simulink model "htx_intent_estimator_base"  (R2024b)
settings: Solver=VariableStepAuto  StartTime=0.0  StopTime=1  FixedStep=0.001  RelTol=1e-3
libraries: simulink_extras x1
settings Model: Creator=lukec  LastModifiedBy=lukec
settings SolverCC: ZeroCrossControl=DisableAll

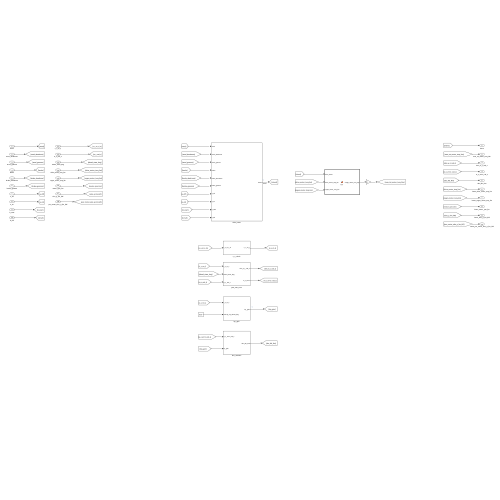
[thumbnail: Simulink's stored preview of the top-level diagram]
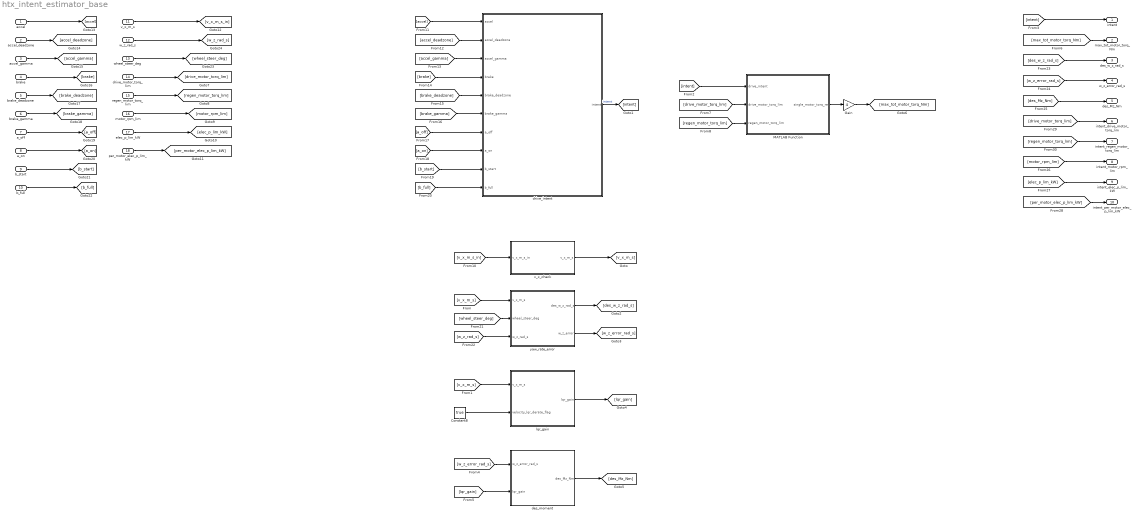
== system htx_intent_estimator_base ==
  accel : Inport
  accel_deadzone : Inport  Port=2
  accel_gamma : Inport  Port=3
  brake : Inport  Port=4
  brake_deadzone : Inport  Port=5
  brake_gamma : Inport  Port=6
  a_off : Inport  Port=7
  a_on : Inport  Port=8
  b_start : Inport  Port=9
  b_full : Inport  Port=10
  v_x_m_s : Inport  Port=11
  w_z_rad_s : Inport  Port=12
  wheel_steer_deg : Inport  Port=13
  drive_motor_torq_lim : Inport  Port=14
  regen_motor_torq_lim : Inport  Port=15
  motor_rpm_lim : Inport  Port=16
  elec_p_lim_kW : Inport  Port=17
  per_motor_elec_p_lim_kW : Inport  Port=18
  Constant8 : Constant  Value=true
  Gain : Gain  Gain=4
  MATLAB Function : MATLAB Function  TreatAsAtomicUnit=on
  des_moment : Subsystem
  drive_intent : Subsystem
  lqr_gain : Subsystem
  v_x_check : Subsystem
  yaw_rate_error : Subsystem
  intent : Outport
  max_tot_motor_torq_Nm : Outport  Port=2
  des_w_z_rad_s : Outport  Port=3
  w_z_error_rad_s : Outport  Port=4
  des_Mz_Nm : Outport  Port=5
  intent_drive_motor_torq_lim : Outport  Port=6
  intent_regen_motor_torq_lim : Outport  Port=7
  intent_motor_rpm_lim : Outport  Port=8
  intent_elec_p_lim_kW : Outport  Port=9
  intent_per_motor_elec_p_lim_kW : Outport  Port=10
  wires:
  Constant8/1 -> lqr_gain/2(velocity_lqr_derate_flag)
  lqr_gain/1(lqr_gain) -> [lqr_gain]
  [v_x_m_s] -> yaw_rate_error/1(v_x_m_s)
  [v_x_m_s] -> lqr_gain/1(v_x_m_s)
  MATLAB Function/1(single_motor_torq_req) -> Gain/1
  drive_intent/1(intent) -> [intent]  "intent"
  [intent] -> MATLAB Function/1(drive_intent)
  [intent] -> intent/1
  yaw_rate_error/1(des_w_z_rad_s) -> [des_w_z_rad_s]
  yaw_rate_error/2(w_z_error) -> [w_z_error_rad_s]
  [w_z_error_rad_s] -> des_moment/1(w_z_error_rad_s)
  [lqr_gain] -> des_moment/2(lqr_gain)
  des_moment/1(des_Mz_Nm) -> [des_Mz_Nm]
  Gain/1 -> [max_tot_motor_torq_Nm]
  [max_tot_motor_torq_Nm] -> max_tot_motor_torq_Nm/1
  regen_motor_torq_lim/1 -> [regen_motor_torq_lim]
  drive_motor_torq_lim/1 -> [drive_motor_torq_lim]
  [drive_motor_torq_lim] -> MATLAB Function/2(drive_motor_torq_lim)
  [regen_motor_torq_lim] -> MATLAB Function/3(regen_motor_torq_lim)
  motor_rpm_lim/1 -> [motor_rpm_lim]
  elec_p_lim_kW/1 -> [elec_p_lim_kW]
  per_motor_elec_p_lim_kW/1 -> [per_motor_elec_p_lim_kW]
  v_x_m_s/1 -> [v_x_m_s_in]
  accel/1 -> [accel]
  accel_deadzone/1 -> [accel_deadzone]
  accel_gamma/1 -> [accel_gamma]
  brake/1 -> [brake]
  brake_deadzone/1 -> [brake_deadzone]
  brake_gamma/1 -> [brake_gamma]
  a_off/1 -> [a_off]
  a_on/1 -> [a_on]
  b_start/1 -> [b_start]
  b_full/1 -> [b_full]
  [accel] -> drive_intent/1(accel)
  [accel_deadzone] -> drive_intent/2(accel_deadzone)
  [accel_gamma] -> drive_intent/3(accel_gamma)
  [b_full] -> drive_intent/10(b_full)
  [b_start] -> drive_intent/9(b_start)
  [a_on] -> drive_intent/8(a_on)
  [a_off] -> drive_intent/7(a_off)
  [brake_gamma] -> drive_intent/6(brake_gamma)
  [brake_deadzone] -> drive_intent/5(brake_deadzone)
  [brake] -> drive_intent/4(brake)
  wheel_steer_deg/1 -> [wheel_steer_deg]
  w_z_rad_s/1 -> [w_z_rad_s]
  [wheel_steer_deg] -> yaw_rate_error/2(wheel_steer_deg)
  [w_z_rad_s] -> yaw_rate_error/3(w_z_rad_s)
  [des_w_z_rad_s] -> des_w_z_rad_s/1
  [w_z_error_rad_s] -> w_z_error_rad_s/1
  [des_Mz_Nm] -> des_Mz_Nm/1
  [motor_rpm_lim] -> intent_motor_rpm_lim/1
  [elec_p_lim_kW] -> intent_elec_p_lim_kW/1
  [per_motor_elec_p_lim_kW] -> intent_per_motor_elec_p_lim_kW/1
  [drive_motor_torq_lim] -> intent_drive_motor_torq_lim/1
  [regen_motor_torq_lim] -> intent_regen_motor_torq_lim/1
  [v_x_m_s_in] -> v_x_check/1(v_x_m_s_in)
  v_x_check/1(v_x_m_s) -> [v_x_m_s]

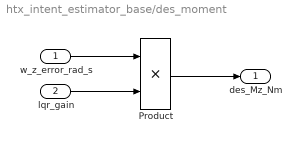
== system htx_intent_estimator_base/des_moment ==
  w_z_error_rad_s : Inport
  lqr_gain : Inport  Port=2
  Product : Product
  des_Mz_Nm : Outport
  wires:
  w_z_error_rad_s/1 -> Product/1
  lqr_gain/1 -> Product/2
  Product/1 -> des_Mz_Nm/1

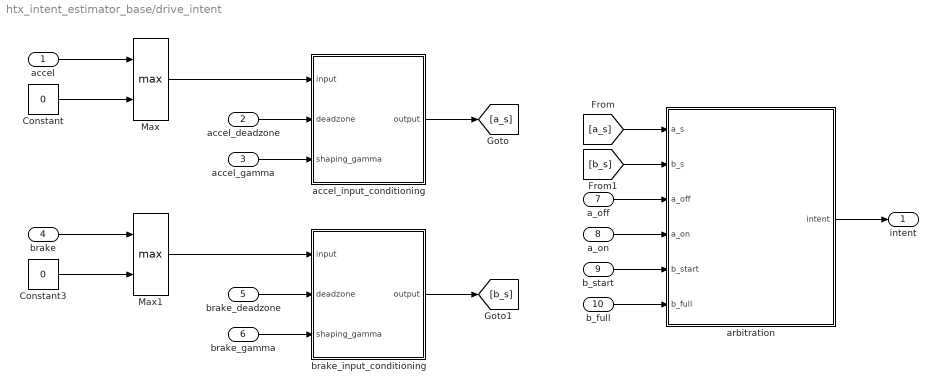
== system htx_intent_estimator_base/drive_intent ==
  accel : Inport
  accel_deadzone : Inport  Port=2
  accel_gamma : Inport  Port=3
  brake : Inport  Port=4
  brake_deadzone : Inport  Port=5
  brake_gamma : Inport  Port=6
  a_off : Inport  Port=7
  a_on : Inport  Port=8
  b_start : Inport  Port=9
  b_full : Inport  Port=10
  Constant : Constant  Value=0
  Constant3 : Constant  Value=0
  Max : MinMax  Function=max  Inputs=2
  Max1 : MinMax  Function=max  Inputs=2
  accel_input_conditioning : Subsystem
  arbitration : Subsystem
  brake_input_conditioning : Subsystem
  intent : Outport
  wires:
  accel/1 -> Max/1
  Constant/1 -> Max/2
  Max/1 -> accel_input_conditioning/1(input)
  accel_gamma/1 -> accel_input_conditioning/3(shaping_gamma)
  accel_input_conditioning/1(output) -> [a_s]
  accel_deadzone/1 -> accel_input_conditioning/2(deadzone)
  brake/1 -> Max1/1
  Constant3/1 -> Max1/2
  Max1/1 -> brake_input_conditioning/1(input)
  brake_deadzone/1 -> brake_input_conditioning/2(deadzone)
  brake_gamma/1 -> brake_input_conditioning/3(shaping_gamma)
  brake_input_conditioning/1(output) -> [b_s]
  [a_s] -> arbitration/1(a_s)
  [b_s] -> arbitration/2(b_s)
  arbitration/1(intent) -> intent/1
  a_off/1 -> arbitration/3(a_off)
  a_on/1 -> arbitration/4(a_on)
  b_start/1 -> arbitration/5(b_start)
  b_full/1 -> arbitration/6(b_full)

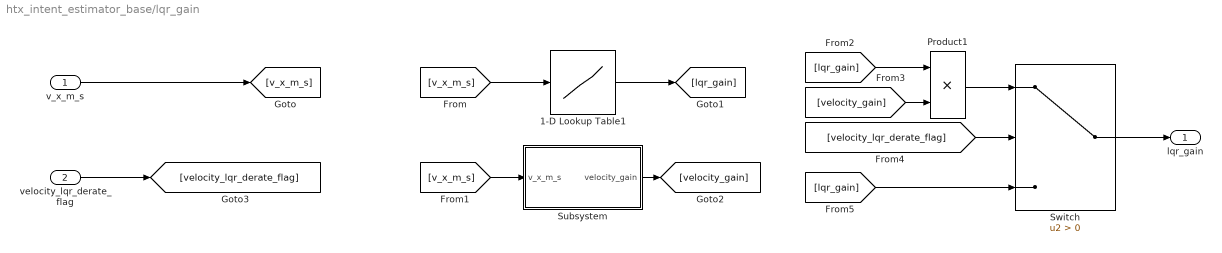
== system htx_intent_estimator_base/lqr_gain ==
  v_x_m_s : Inport
  velocity_lqr_derate_flag : Inport  Port=2
  1-D Lookup Table1 : Lookup_n-D  NumberOfTableDimensions=1  BreakpointsForDimension1="[1\t2\t3\t4\t5\t6\t7\t8\t9\t10\t11\t12\t13\t14\t15\t16\t17\t18\t19\t20\t21\t22\t23\t24\t25\t26\t27\t28\t29\t30\t31\t32\t33\t34\t35]"  Table=|  ExtrapMethod=Clip  UseLastTableValue=on  InternalRulePriority=Speed  RndMeth=Simplest
      | [175.998769578400
      | 348.795608426570
      | 515.559078921668
      | 674.093445795412
      | 822.946224394498
      | 961.371891615202
      | 1089.20563526030
      | 1206.70525770109
      | 1314.40207126520
      | 1412.98049731322
      | 1503.19064596410
      | 1585.79003907249
      | 1661.50785065425
      | 1731.02511425824
      | 1794.96555127361
      | 1853.89307906945
      | 1908.31327556636
      | 1958.67700477001
      | 2005.38506538649
      | 2048.79316923418
      | 2089.21684666341
      | 2126.93606072781
      | 2162.19942593451
      | 2195.22799578584
      | 2226.21862266091
      | 2255.34691480485
      | 2282.76982535041
      | 2308.62791187574
      | 2333.04730481808
      | 2356.14142085417
      | 2378.01245418101
      | 2398.75267510957
      | 2418.44556187634
      | 2437.16678827469
      | 2454.98508670055]
  Product1 : Product
  Subsystem : Subsystem
  Switch : Switch  Criteria=u2 > Threshold  SaturateOnIntegerOverflow=off  InputSameDT=off
  lqr_gain : Outport
  wires:
  Product1/1 -> Switch/1
  v_x_m_s/1 -> [v_x_m_s]
  [v_x_m_s] -> 1-D Lookup Table1/1
  1-D Lookup Table1/1 -> [lqr_gain]
  [v_x_m_s] -> Subsystem/1(v_x_m_s)
  Subsystem/1(velocity_gain) -> [velocity_gain]
  [lqr_gain] -> Product1/1
  [velocity_gain] -> Product1/2
  velocity_lqr_derate_flag/1 -> [velocity_lqr_derate_flag]
  [velocity_lqr_derate_flag] -> Switch/2
  [lqr_gain] -> Switch/3
  Switch/1 -> lqr_gain/1

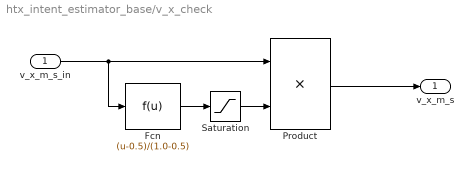
== system htx_intent_estimator_base/v_x_check ==
  v_x_m_s_in : Inport
  Fcn : Fcn  Expr=(u-0.5)/(1.0-0.5)
  Product : Product
  Saturation : Saturate  UpperLimit=1  LowerLimit=0
  v_x_m_s : Outport
  wires:
  v_x_m_s_in/1 -> Fcn/1, Product/1
  Product/1 -> v_x_m_s/1
  Fcn/1 -> Saturation/1
  Saturation/1 -> Product/2

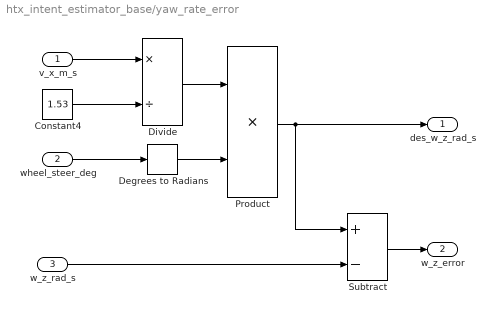
== system htx_intent_estimator_base/yaw_rate_error ==
  v_x_m_s : Inport
  wheel_steer_deg : Inport  Port=2
  w_z_rad_s : Inport  Port=3
  Constant4 : Constant  Value=1.53
  Degrees to Radians : simulink_extras/Transformations/Degrees to Radians
  Divide : Product  Inputs=*/
  Product : Product
  Subtract : Sum  Inputs=+-
  des_w_z_rad_s : Outport
  w_z_error : Outport  Port=2
  wires:
  wheel_steer_deg/1 -> Degrees to Radians/1
  Divide/1 -> Product/1
  Degrees to Radians/1 -> Product/2
  Constant4/1 -> Divide/2
  v_x_m_s/1 -> Divide/1
  Product/1 -> des_w_z_rad_s/1, Subtract/1
  w_z_rad_s/1 -> Subtract/2
  Subtract/1 -> w_z_error/1

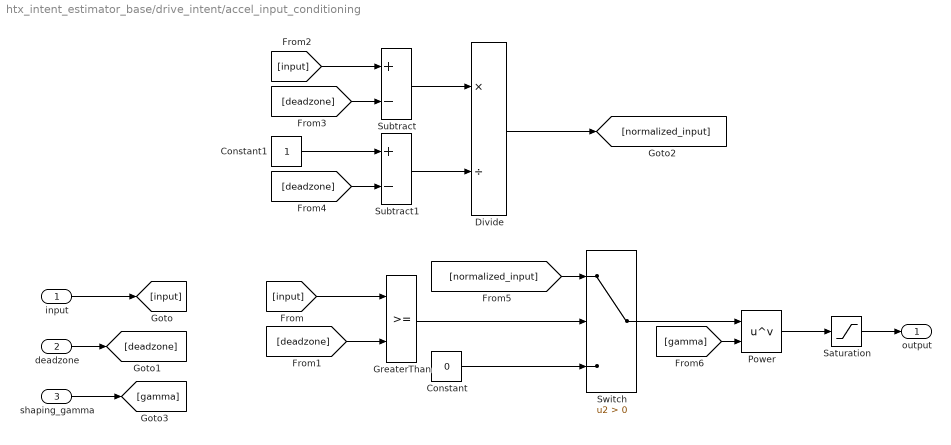
== system htx_intent_estimator_base/drive_intent/accel_input_conditioning ==
  input : Inport
  deadzone : Inport  Port=2
  shaping_gamma : Inport  Port=3
  Constant : Constant  Value=0
  Constant1 : Constant
  Divide : Product  Inputs=*/
  GreaterThan : RelationalOperator  OutDataTypeStr=boolean  RndMeth=Simplest  InputSameDT=off
  Power : Math  Operator=pow
  Saturation : Saturate  UpperLimit=1  LowerLimit=0
  Subtract : Sum  Inputs=+-
  Subtract1 : Sum  Inputs=+-
  Switch : Switch  Criteria=u2 > Threshold  SaturateOnIntegerOverflow=off  InputSameDT=off
  output : Outport
  wires:
  GreaterThan/1 -> Switch/2
  Constant/1 -> Switch/3
  input/1 -> [input]
  deadzone/1 -> [deadzone]
  [input] -> GreaterThan/1
  [deadzone] -> GreaterThan/2
  [input] -> Subtract/1
  [deadzone] -> Subtract/2
  Subtract/1 -> Divide/1
  Constant1/1 -> Subtract1/1
  [deadzone] -> Subtract1/2
  Subtract1/1 -> Divide/2
  Divide/1 -> [normalized_input]
  [normalized_input] -> Switch/1
  shaping_gamma/1 -> [gamma]
  Switch/1 -> Power/1
  [gamma] -> Power/2
  Power/1 -> Saturation/1
  Saturation/1 -> output/1

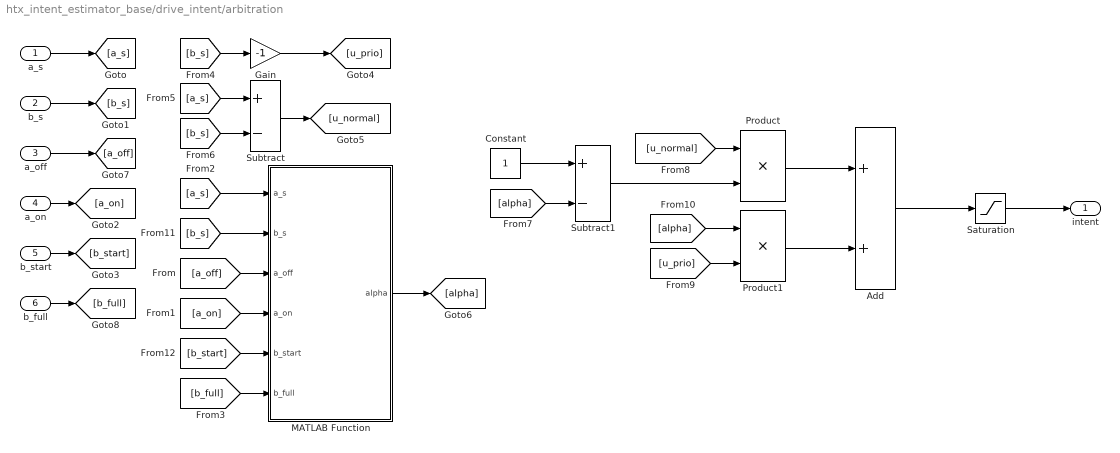
== system htx_intent_estimator_base/drive_intent/arbitration ==
  a_s : Inport
  b_s : Inport  Port=2
  a_off : Inport  Port=3
  a_on : Inport  Port=4
  b_start : Inport  Port=5
  b_full : Inport  Port=6
  Add : Sum
  Constant : Constant
  Gain : Gain  Gain=-1
  MATLAB Function : MATLAB Function  TreatAsAtomicUnit=on
  Product : Product
  Product1 : Product
  Saturation : Saturate  UpperLimit=1  LowerLimit=-1
  Subtract : Sum  Inputs=+-
  Subtract1 : Sum  Inputs=+-
  intent : Outport
  wires:
  a_s/1 -> [a_s]
  b_s/1 -> [b_s]
  b_start/1 -> [b_start]
  [b_s] -> Gain/1
  Gain/1 -> [u_prio]
  [a_s] -> Subtract/1
  [b_s] -> Subtract/2
  Subtract/1 -> [u_normal]
  Saturation/1 -> intent/1
  Constant/1 -> Subtract1/1
  [alpha] -> Subtract1/2
  Subtract1/1 -> Product/2
  [u_normal] -> Product/1
  [u_prio] -> Product1/2
  [alpha] -> Product1/1
  Product/1 -> Add/1
  Product1/1 -> Add/2
  MATLAB Function/1(alpha) -> [alpha]
  Add/1 -> Saturation/1
  a_on/1 -> [a_on]
  b_full/1 -> [b_full]
  [b_s] -> MATLAB Function/2(b_s)
  [a_s] -> MATLAB Function/1(a_s)
  [a_off] -> MATLAB Function/3(a_off)
  [b_start] -> MATLAB Function/5(b_start)
  [b_full] -> MATLAB Function/6(b_full)
  a_off/1 -> [a_off]
  [a_on] -> MATLAB Function/4(a_on)

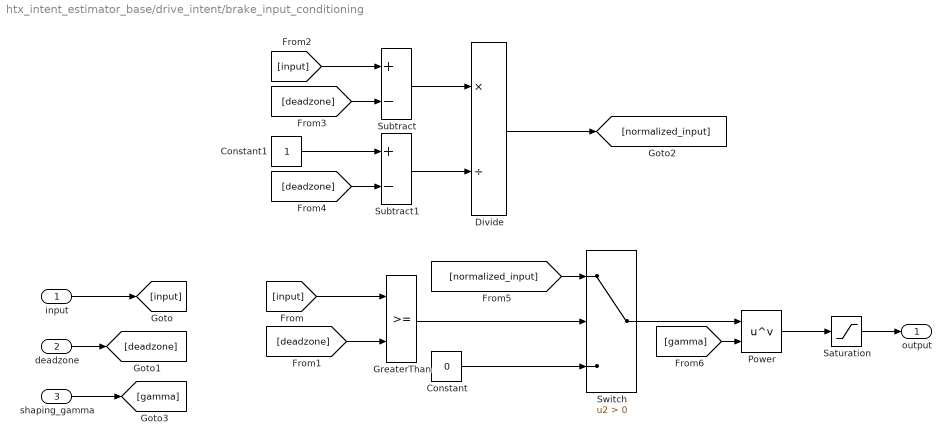
== system htx_intent_estimator_base/drive_intent/brake_input_conditioning ==
  input : Inport
  deadzone : Inport  Port=2
  shaping_gamma : Inport  Port=3
  Constant : Constant  Value=0
  Constant1 : Constant
  Divide : Product  Inputs=*/
  GreaterThan : RelationalOperator  OutDataTypeStr=boolean  RndMeth=Simplest  InputSameDT=off
  Power : Math  Operator=pow
  Saturation : Saturate  UpperLimit=1  LowerLimit=0
  Subtract : Sum  Inputs=+-
  Subtract1 : Sum  Inputs=+-
  Switch : Switch  Criteria=u2 > Threshold  SaturateOnIntegerOverflow=off  InputSameDT=off
  output : Outport
  wires:
  Saturation/1 -> output/1
  Power/1 -> Saturation/1
  [gamma] -> Power/2
  Switch/1 -> Power/1
  shaping_gamma/1 -> [gamma]
  [normalized_input] -> Switch/1
  Divide/1 -> [normalized_input]
  Subtract1/1 -> Divide/2
  [deadzone] -> Subtract1/2
  Constant1/1 -> Subtract1/1
  Subtract/1 -> Divide/1
  [deadzone] -> Subtract/2
  [input] -> Subtract/1
  [deadzone] -> GreaterThan/2
  [input] -> GreaterThan/1
  deadzone/1 -> [deadzone]
  input/1 -> [input]
  Constant/1 -> Switch/3
  GreaterThan/1 -> Switch/2

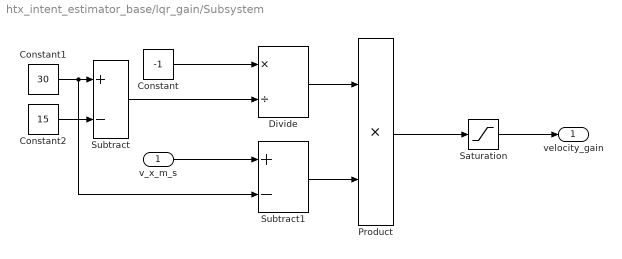
== system htx_intent_estimator_base/lqr_gain/Subsystem ==
  v_x_m_s : Inport
  Constant : Constant  Value=-1
  Constant1 : Constant  Value=30
  Constant2 : Constant  Value=15
  Divide : Product  Inputs=*/
  Product : Product
  Saturation : Saturate  UpperLimit=1  LowerLimit=0
  Subtract : Sum  Inputs=+-
  Subtract1 : Sum  Inputs=+-
  velocity_gain : Outport
  wires:
  Subtract1/1 -> Product/2
  Product/1 -> Saturation/1
  Constant2/1 -> Subtract/2
  Constant/1 -> Divide/1
  Subtract/1 -> Divide/2
  Divide/1 -> Product/1
  Constant1/1 -> Subtract1/2, Subtract/1
  v_x_m_s/1 -> Subtract1/1
  Saturation/1 -> velocity_gain/1

== matlab function htx_intent_estimator_base/MATLAB Function ==
  data: drive_intent input; single_motor_torq_req output; drive_motor_torq_lim input; regen_motor_torq_lim input
function single_motor_torq_req = fcn(drive_intent, drive_motor_torq_lim, regen_motor_torq_lim)

    if drive_intent == 0
        single_motor_torq_req = 0;
    elseif drive_intent < 0
        single_motor_torq_req = interp1([-1 0], [regen_motor_torq_lim, 0], drive_intent);
    else
        single_motor_torq_req = interp1([0 1], [0, drive_motor_torq_lim], drive_intent);
    end

== matlab function htx_intent_estimator_base/drive_intent/arbitration/MATLAB Function ==
  data: a_s input; b_s input; alpha output; a_off input; a_on input; b_start input; b_full input
function alpha = fcn(a_s, b_s, a_off, a_on, b_start, b_full)

% Brake-based alpha
if b_s <= b_start
    alpha_b = 0;
elseif b_s >= b_full
    alpha_b = 1;
else
    alpha_b = (b_s - b_start) / (b_full - b_start);
end

% Smooth throttle gate
if a_s <= a_off
    g = 0;
elseif a_s >= a_on
    g = 1;
else
    g = (a_s - a_off) / (a_on - a_off);
end

alpha = alpha_b * g;
alpha = min(max(alpha,0),1);
